simulink model "PMSM_PLL0707"  (R2018b)
settings: Solver=ode45  StartTime=0.0  StopTime=15  FixedStep=Ts  RelTol=1e-4  EnableMultiTasking=on
InitFcn:
  | Ts = 1e-5;
  | Tsample = 1e-3;
  | 
  | Rs = 0.8975;
  | Ld = 1.5e-3;
  | Lq = 1.5e-3;
  | Pn = 3;
  | flux = 0.1764;
  | 
  | Kp_PLL = 1500;
  | Ki_PLL = 1000;
undefined symbols (not defined in the file): DiscIntNeverNeededParam
libraries: powerlib x5, powerlib_extras x2, simulink x1
settings Model: Creator=SUN  LastModifiedBy=liangjin
settings SolverCC: ZeroCrossControl=DisableAll
settings DataIOCC: LimitDataPoints=on  SaveFormat=Array
settings OptimizationCC: ExpressionDepthLimit=2147483647  InitFltsAndDblsToZero=on  LifeSpan=inf
settings DebuggingCC: UnderspecifiedInitializationDetection=Classic  MergeDetectMultiDrivingBlocksExec=none  SolverPrmCheckMsg=warning  FcnCallInpInsideContextMsg=warning  StateNameClashWarn=warning  SFUnexpectedBacktrackingDiag=warning  SFNoUnconditionalDefaultTransitionDiag=warning  SFExecutionAtInitializationDiag=none
settings HardwareCC: ProdBitPerPointer=32  ProdBitPerSizeT=32  ProdBitPerPtrDiffT=32  ProdLargestAtomicFloat=None  ProdIntDivRoundTo=Undefined  ProdEndianess=Unspecified  ProdWordSize=32  ProdHWDeviceType=32-bit Generic
settings ModelReferenceCC: PropagateSignalLabelsOutOfModel=off
settings SFSimCC: SimUseLocalCustomCode=off
settings RTWCC: RTWUseLocalCustomCode=off
settings CodeAppCC: StateflowObjectComments=on
settings GRTTargetCC: TargetLangStandard=C89/C90 (ANSI)  GeneratePreprocessorConditionals=Disable all  CombineOutputUpdateFcns=off  GRTInterface=on
settings ConfigComp: CovMetricSettings=dw  CovHtmlReporting=on  CovSaveCumulativeToWorkspaceVar=on  CovSaveSingleToWorkspaceVar=on  CovExternalEMLEnable=off  CovSFcnEnable=off
settings SimscapeCC: SimscapeNormalizeSystem=off

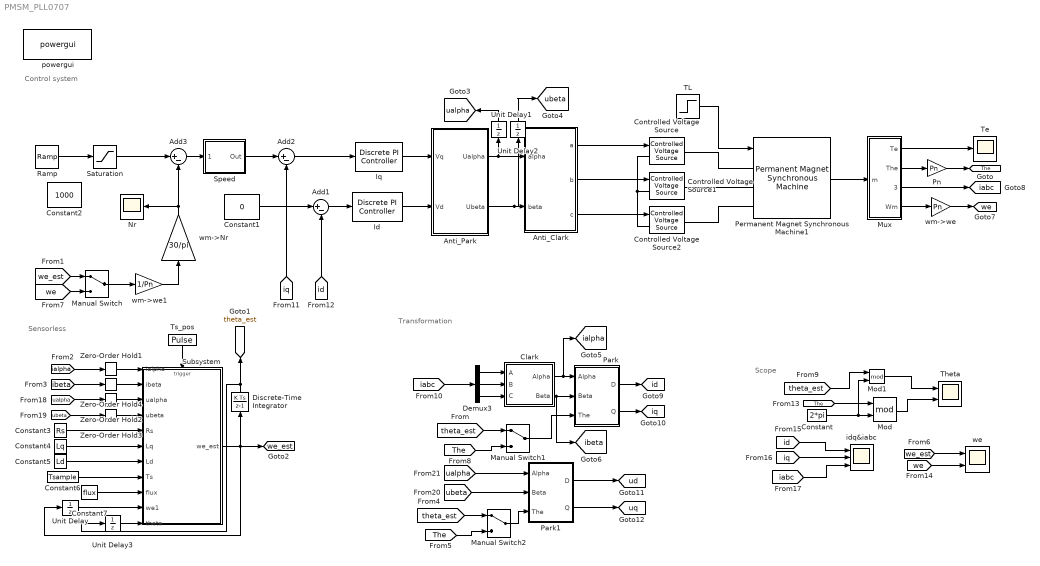
== system PMSM_PLL0707 ==
  note: Scope
  note: Control system
  note: Transformation
  note: Sensorless
  Add1 : Sum  Inputs=|+-
  Add2 : Sum  Inputs=|+-
  Add3 : Sum  Inputs=|+-
  Anti_Clark : Subsystem
  Anti_Park : Subsystem
  Clark : Subsystem
  Constant : Constant  Value=2*pi
  Constant1 : Constant  Value=0
  Constant2 : Constant  Value=1000
  Constant3 : Constant  Value=Rs
  Constant4 : Constant  Value=Lq
  Constant5 : Constant  Value=Ld
  Constant6 : Constant  Value=Tsample
  Constant7 : Constant  Value=flux
  Controlled Voltage Source : powerlib/Electrical Sources/Controlled Voltage Source  Initialize=on  Source_Type=AC  Amplitude=0  Phase=0  Frequency=0  Measurements=None
      settings: SourceProductName=Simscape Electrical
  Controlled Voltage Source1 : powerlib/Electrical Sources/Controlled Voltage Source  Initialize=on  Source_Type=AC  Amplitude=0  Phase=0  Frequency=0  Measurements=None
      settings: SourceProductName=Simscape Electrical
  Controlled Voltage Source2 : powerlib/Electrical Sources/Controlled Voltage Source  Initialize=on  Source_Type=AC  Amplitude=0  Phase=0  Frequency=0  Measurements=None
      settings: SourceProductName=Simscape Electrical
  Demux3 : Demux  Outputs=3
  Discrete-Time Integrator : DiscreteIntegrator  gainval=1  SampleTime=Ts  ICPrevOutput=DiscIntNeverNeededParam  ICPrevScaledInput=DiscIntNeverNeededParam
  Id : powerlib_extras/Discrete  Control Blocks/Discrete PI Controller  Kp=Ld*376  Ki=Rs*376  Par_Limits=[311*0.9*sqrt(1/3) -311*0.9*sqrt(1/3)]  Init=0  Ts=Ts*10
  Iq : powerlib_extras/Discrete  Control Blocks/Discrete PI Controller  Kp=Lq*376  Ki=Rs*376  Par_Limits=[311*0.9*sqrt(1/3) -311*0.9*sqrt(1/3)]  Init=0  Ts=Ts*10
  Manual Switch : ManualSwitch
  Manual Switch1 : ManualSwitch
  Manual Switch2 : ManualSwitch
  Mod : Math  Operator=mod  SaturateOnIntegerOverflow=on
  Mod1 : Math  Operator=mod  SaturateOnIntegerOverflow=on
  Mux : Subsystem
  Nr : Scope
  Park : Subsystem
  Park1 : Subsystem
  Permanent Magnet Synchronous Machine1 : powerlib/Machines/Permanent Magnet Synchronous Machine  NbPhases=3  FluxDistribution=Sinusoidal  RotorType=Salient-pole  MechanicalLoad=Torque Tm  PresetModel=No  ShowDetailedParameters=on  MeasurementBus=off  Resistance=0.8975  Inductance=8.5e-3  dqInductances=[1.5e-3,1.5e-3]  La=0.000835  MachineConstant=Flux linkage established by magnets (V.s)  Flux=0.1764  VoltageCst=95.9863  TorqueCst=0.7938  Flat=120  Mechanical=[0.000311 0.0000001 3]  PolePairs=3  InitialConditions=[0,0, 0,0]  InitialConditions5ph=[0 0 0 0 0 0]  TsPowergui=0  TsBlock=-1  RefAngle=Aligned with phase A axis (original Park)
  Pn : Gain  Gain=Pn
  Ramp : simulink/Sources/Ramp  slope=500  start=0  InitialOutput=0
  Saturation : Saturate  UpperLimit=1000  LowerLimit=-1000
  Speed : Subsystem  AncestorBlock=|  DialogController=POWERSYS.PowerSysDialog  mask(Discrete PI Controller){Kpw=0.01, Kiw=0.01*50, Ba=0, Par_Limits=[80 -80], Init=0, Ts=100*Ts}
      | powerlib_extras/Discrete 
      | Control Blocks/Discrete
      | PI Controller
      mask prompts: Kpw "Proportional gain (Kp):"; Kiw "Integral gain (Ki):"; Ba "feedback gain (Ba)"; Par_Limits "Output limits: [ Upper   Lower ]"; Init "Output initial value:"; Ts "Sample time:"
      mask help: This block implements a discrete PI controller.
      mask init:
      | UpperLimit=Par_Limits(1);
      | LowerLimit=Par_Limits(2);
      | power_initmask();
      mask Help: This block is part of a subset of blocks in the Extras library that does not have documentation associated with it, other than the block mask description.
      mask Display: disp('PI');
  Subsystem : Subsystem
  TL : Step  Time=0  After=0  SampleTime=Ts
  Te : Scope
  Theta : Scope  NumInputPorts=2
  Ts_pos : DiscretePulseGenerator  PulseType=Time based  Period=1e-3  PulseWidth=50
  Unit Delay : UnitDelay  SampleTime=-1
  Unit Delay1 : UnitDelay  SampleTime=10*Ts
  Unit Delay2 : UnitDelay  SampleTime=10*Ts
  Unit Delay3 : UnitDelay  SampleTime=-1
  Zero-Order Hold{1..4} (4 alike) : ZeroOrderHold  SampleTime=10*Ts
  idq&iabc : Scope  NumInputPorts=3
  powergui : powerlib/powergui  SimulationMode=Discrete  SampleTime=Ts  frequency=60  Iterations=50  frequencyindice=0  Pbase=100e6  ErrMax=1e-4  UnitsV=kV  UnitsW=MW  buscounter=0  FunctionMessages=off  echomessages=off  EnableUseOfTLC=off  CurrentSourceSwitches=off  DisableSnubberDevices=off  DisableRonSwitches=off  DisableVfSwitches=off  DisplayEquations=off  SolverType=Tustin/Backward Euler (TBE)  Interpol=off  ExternalGateDelay=off  methode=off  Ts=100  x0status=blocks  SPID=off  SwTol=0  HookPort=off  RestoreLinks=warning  ResistiveCurrentMeasurement=off  Frange=[0:2:500]  Ylog=off  Xlog=on  ShowGrid=off  save=off  variable=ZData  structure=0  ZoomFFT=on  StartTime=0.0  cycles=1  DisplayStyle=1  fundamental=60  FreqAxis=off  MaxFrequency=1000  frequencyindicesteady=1  RmsSteady=1  display=off
  we : Scope  NumInputPorts=2
  wm->Nr : Gain  Gain=30/pi
  wm->we : Gain  Gain=Pn
  wm->we1 : Gain  Gain=1/Pn
  tag scope: The=global, iabc=global, ialpha=global, ibeta=global, id=global, iq=global, theta_est=global, ualpha=global, ubeta=global, ud=global, uq=global, we=global, we_est=global
  wires:
  TL/1 -> Permanent Magnet Synchronous Machine1/1
  Permanent Magnet Synchronous Machine1/1 -> Mux/1(m)
  Add3/1 -> Speed/1(Error)
  Constant1/1 -> Add1/1
  Add1/1 -> Id/1
  wm->Nr/1 -> Add3/2, Nr/1
  Add2/1 -> Iq/1
  Mux/1(Te) -> Te/1
  Mux/2(The) -> Pn/1
  Pn/1 -> [The]
  Mux/4(Wm) -> wm->we/1
  Mux/3(Iabc) -> [iabc]
  Clark/1(Alpha) -> [ialpha], Park/1(Alpha)
  Demux3/1 -> Clark/1(A)
  Demux3/2 -> Clark/2(B)
  Demux3/3 -> Clark/3(C)
  Clark/2(Beta) -> Park/2(Beta), [ibeta]
  Iq/1 -> Anti_Park/1(Vq)
  Id/1 -> Anti_Park/2(Vd)
  Anti_Clark/1(a) -> Controlled Voltage Source/1
  Anti_Clark/2(b) -> Controlled Voltage Source1/1
  Anti_Clark/3(c) -> Controlled Voltage Source2/1
  Speed/1(Out) -> Add2/1
  Constant/1 -> Mod/2, Mod1/2
  Mod/1 -> Theta/2
  wm->we/1 -> [we]
  Ramp/1 -> Saturation/1
  wm->we1/1 -> wm->Nr/1
  Anti_Park/1(Ualpha) -> Unit Delay1/1, Anti_Clark/1(alpha)
  Anti_Park/2(Ubeta) -> Unit Delay2/1, Anti_Clark/2(beta)
  [we_est] -> we/1
  [we_est] -> Manual Switch/1
  [we] -> Manual Switch/2
  [theta_est] -> Manual Switch1/1
  Manual Switch1/1 -> Park/3(The)
  [The] -> Manual Switch1/2
  Saturation/1 -> Add3/1
  [iabc] -> Demux3/1
  Park/1(D) -> [id]
  Park/2(Q) -> [iq]
  [The] -> Mod/1
  [we] -> we/2
  [id] -> idq&iabc/1
  [iq] -> idq&iabc/2
  [iabc] -> idq&iabc/3
  [id] -> Add1/2
  [iq] -> Add2/2
  Manual Switch/1 -> wm->we1/1
  [ualpha] -> Zero-Order Hold2/1
  [ubeta] -> Zero-Order Hold3/1
  [ialpha] -> Zero-Order Hold1/1
  [ibeta] -> Zero-Order Hold4/1
  [The] -> Manual Switch2/2
  Manual Switch2/1 -> Park1/3(The)
  [theta_est] -> Manual Switch2/1
  [ubeta] -> Park1/2(Beta)
  [ualpha] -> Park1/1(Alpha)
  Park1/1(D) -> [ud]
  Park1/2(Q) -> [uq]
  Unit Delay1/1 -> [ualpha]
  Unit Delay2/1 -> [ubeta]
  Discrete-Time Integrator/1 -> [theta_est], Unit Delay3/1
  Subsystem/1(we_est) -> Discrete-Time Integrator/1, [we_est], Unit Delay/1
  Zero-Order Hold1/1 -> Subsystem/1(ialpha)
  Zero-Order Hold4/1 -> Subsystem/2(ibeta)
  Zero-Order Hold2/1 -> Subsystem/3(ualpha)
  Zero-Order Hold3/1 -> Subsystem/4(ubeta)
  Constant3/1 -> Subsystem/5(Rs)
  Constant4/1 -> Subsystem/6(Lq)
  Constant5/1 -> Subsystem/7(Ld)
  Constant6/1 -> Subsystem/8(Ts)
  Constant7/1 -> Subsystem/9(flux)
  Unit Delay/1 -> Subsystem/10(we1)
  Ts_pos/1 -> Subsystem/Trigger
  Unit Delay3/1 -> Subsystem/11(theta)
  [theta_est] -> Mod1/1
  Mod1/1 -> Theta/1
  connections:
  Controlled Voltage Source/LConn1 -- Controlled Voltage Source2/LConn1 -- Controlled Voltage Source1/LConn1
  Controlled Voltage Source/RConn1 -- Permanent Magnet Synchronous Machine1/LConn1
  Controlled Voltage Source1/RConn1 -- Permanent Magnet Synchronous Machine1/LConn2
  Controlled Voltage Source2/RConn1 -- Permanent Magnet Synchronous Machine1/LConn3

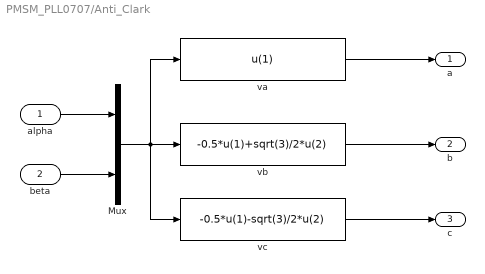
== system PMSM_PLL0707/Anti_Clark ==
  alpha : Inport
  beta : Inport  Port=2
  Mux : Mux  Inputs=2
  va : Fcn  Expr=u(1)
  vb : Fcn  Expr=-0.5*u(1)+sqrt(3)/2*u(2)
  vc : Fcn  Expr=-0.5*u(1)-sqrt(3)/2*u(2)
  a : Outport
  b : Outport  Port=2
  c : Outport  Port=3
  wires:
  va/1 -> a/1
  beta/1 -> Mux/2
  alpha/1 -> Mux/1
  Mux/1 -> vc/1, vb/1, va/1
  vb/1 -> b/1
  vc/1 -> c/1

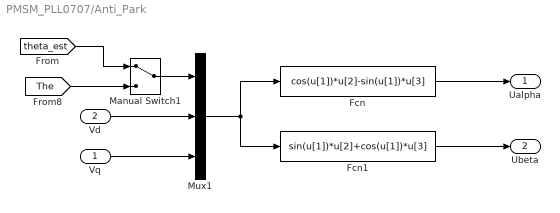
== system PMSM_PLL0707/Anti_Park ==
  Vq : Inport
  Vd : Inport  Port=2
  Fcn : Fcn  Expr=cos(u[1])*u[2]-sin(u[1])*u[3]
  Fcn1 : Fcn  Expr=sin(u[1])*u[2]+cos(u[1])*u[3]
  Manual Switch1 : ManualSwitch
  Mux1 : Mux  Inputs=3
  Ualpha : Outport
  Ubeta : Outport  Port=2
  wires:
  Fcn1/1 -> Ubeta/1
  Fcn/1 -> Ualpha/1
  Mux1/1 -> Fcn/1, Fcn1/1
  Vd/1 -> Mux1/2
  Vq/1 -> Mux1/3
  Manual Switch1/1 -> Mux1/1
  [The] -> Manual Switch1/2
  [theta_est] -> Manual Switch1/1

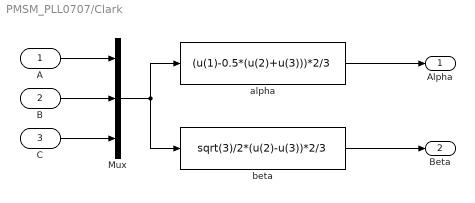
== system PMSM_PLL0707/Clark ==
  A : Inport
  B : Inport  Port=2
  C : Inport  Port=3
  Mux : Mux  Inputs=3
  alpha : Fcn  Expr=(u(1)-0.5*(u(2)+u(3)))*2/3
  beta : Fcn  Expr=sqrt(3)/2*(u(2)-u(3))*2/3
  Alpha : Outport
  Beta : Outport  Port=2
  wires:
  alpha/1 -> Alpha/1
  B/1 -> Mux/2
  C/1 -> Mux/3
  A/1 -> Mux/1
  Mux/1 -> beta/1, alpha/1
  beta/1 -> Beta/1

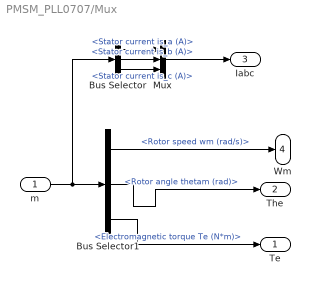
== system PMSM_PLL0707/Mux ==
  m : Inport
  Bus Selector : BusSelector  OutputSignals=Stator current is_a (A),Stator current is_b (A),Stator current is_c (A)
  Bus Selector1 : BusSelector  OutputSignals=Rotor speed wm (rad/s),Rotor angle thetam (rad),Electromagnetic torque Te (N*m)
  Mux : Mux  Inputs=3
  Te : Outport
  The : Outport  Port=2
  Iabc : Outport  Port=3
  Wm : Outport  Port=4
  wires:
  Bus Selector1/1 -> Wm/1  "<Rotor speed wm (rad/s)>"
  Bus Selector1/2 -> The/1  "<Rotor angle thetam (rad)>"
  Bus Selector1/3 -> Te/1  "<Electromagnetic torque Te (N*m)>"
  m/1 -> Bus Selector/1, Bus Selector1/1
  Bus Selector/2 -> Mux/2  "<Stator current is_b (A)>"
  Bus Selector/3 -> Mux/3  "<Stator current is_c (A)>"
  Bus Selector/1 -> Mux/1  "<Stator current is_a (A)>"
  Mux/1 -> Iabc/1

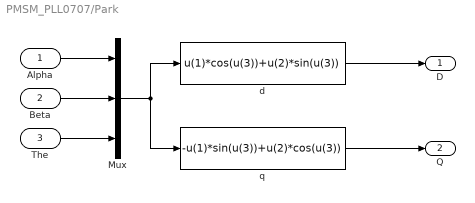
== system PMSM_PLL0707/Park ==
  Alpha : Inport
  Beta : Inport  Port=2
  The : Inport  Port=3
  Mux : Mux  Inputs=3
  d : Fcn  Expr=u(1)*cos(u(3))+u(2)*sin(u(3))
  q : Fcn  Expr=-u(1)*sin(u(3))+u(2)*cos(u(3))
  D : Outport
  Q : Outport  Port=2
  wires:
  d/1 -> D/1
  Beta/1 -> Mux/2
  Alpha/1 -> Mux/1
  Mux/1 -> q/1, d/1
  q/1 -> Q/1
  The/1 -> Mux/3

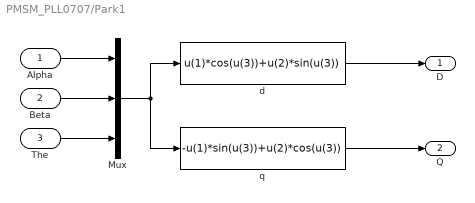
== system PMSM_PLL0707/Park1 ==
  Alpha : Inport
  Beta : Inport  Port=2
  The : Inport  Port=3
  Mux : Mux  Inputs=3
  d : Fcn  Expr=u(1)*cos(u(3))+u(2)*sin(u(3))
  q : Fcn  Expr=-u(1)*sin(u(3))+u(2)*cos(u(3))
  D : Outport
  Q : Outport  Port=2
  wires:
  d/1 -> D/1
  Beta/1 -> Mux/2
  Alpha/1 -> Mux/1
  Mux/1 -> q/1, d/1
  q/1 -> Q/1
  The/1 -> Mux/3

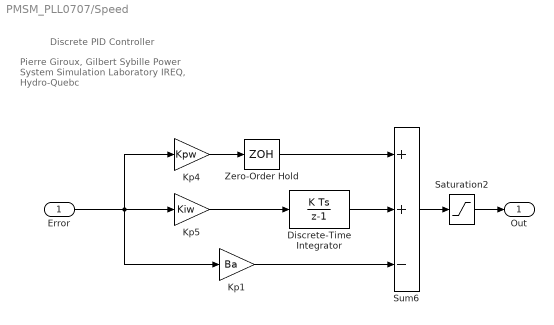
== system PMSM_PLL0707/Speed ==
  note: Discrete PID Controller
  note: Pierre Giroux, Gilbert Sybille
      | Power System Simulation Laboratory
      | IREQ, Hydro-Quebc
  Error : Inport  SampleTime=Ts
  Discrete-Time Integrator : DiscreteIntegrator  InitialCondition=Init  SampleTime=Ts  LimitOutput=on  UpperSaturationLimit=UpperLimit  LowerSaturationLimit=LowerLimit  ICPrevOutput=DiscIntNeverNeededParam  ICPrevScaledInput=DiscIntNeverNeededParam
  Kp1 : Gain  Gain=Ba  SampleTime=Ts  SaturateOnIntegerOverflow=on  OutDataTypeStr=Inherit: Same as input  ParamDataTypeStr=Inherit: Same as input
  Kp4 : Gain  Gain=Kpw  SampleTime=Ts  SaturateOnIntegerOverflow=on  OutDataTypeStr=Inherit: Same as input  ParamDataTypeStr=Inherit: Same as input
  Kp5 : Gain  Gain=Kiw  SampleTime=Ts  SaturateOnIntegerOverflow=on  OutDataTypeStr=Inherit: Same as input  ParamDataTypeStr=Inherit: Same as input
  Saturation2 : Saturate  UpperLimit=UpperLimit  LowerLimit=LowerLimit  SampleTime=Ts
  Sum6 : Sum  Inputs=++-  SampleTime=Ts  SaturateOnIntegerOverflow=on  InputSameDT=on  OutDataTypeStr=Inherit: Same as first input
  Zero-Order Hold : ZeroOrderHold  SampleTime=Ts
  Out : Outport  SampleTime=Ts  InitialOutput=0
  wires:
  Error/1 -> Kp1/1, Kp5/1, Kp4/1
  Zero-Order Hold/1 -> Sum6/1
  Saturation2/1 -> Out/1
  Discrete-Time Integrator/1 -> Sum6/2
  Kp4/1 -> Zero-Order Hold/1
  Kp5/1 -> Discrete-Time Integrator/1
  Sum6/1 -> Saturation2/1
  Kp1/1 -> Sum6/3

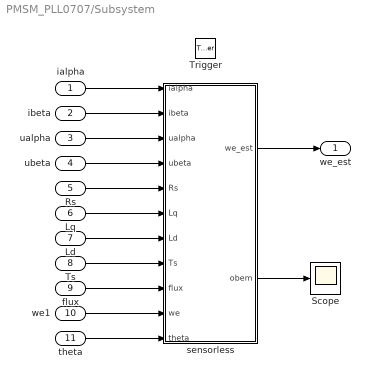
== system PMSM_PLL0707/Subsystem ==
  ialpha : Inport
  ibeta : Inport  Port=2
  ualpha : Inport  Port=3
  ubeta : Inport  Port=4
  Rs : Inport  Port=5
  Lq : Inport  Port=6
  Ld : Inport  Port=7
  Ts : Inport  Port=8
  flux : Inport  Port=9
  we1 : Inport  Port=10
  theta : Inport  Port=11
  Trigger : TriggerPort  VariantControl=Variant  PortDimensions=1
  Scope : Scope
  sensorless : MATLAB Function  TreatAsAtomicUnit=on
  we_est : Outport
  wires:
  ualpha/1 -> sensorless/3(ualpha)
  Ts/1 -> sensorless/8(Ts)
  flux/1 -> sensorless/9(flux)
  ialpha/1 -> sensorless/1(ialpha)
  sensorless/1(we_est) -> we_est/1
  Lq/1 -> sensorless/6(Lq)
  ubeta/1 -> sensorless/4(ubeta)
  ibeta/1 -> sensorless/2(ibeta)
  Rs/1 -> sensorless/5(Rs)
  Ld/1 -> sensorless/7(Ld)
  we1/1 -> sensorless/10(we)
  theta/1 -> sensorless/11(theta)
  sensorless/2(obem) -> Scope/1

== matlab function PMSM_PLL0707/Subsystem/sensorless ==
  data: ialpha input; we_est output; ibeta input; ualpha input; ubeta input; Rs input; Lq input; Ld input; Ts input; flux input; we input; theta input; obem output
function [we_est, obem]  = sensorless(ialpha,ibeta,ualpha,ubeta,Rs,Lq,Ld,Ts,flux,we,theta)

persistent id2 iq2 delta_id delta_iq bemf we1 flag;

if isempty(id2)
    id2=0;iq2=0;delta_id=0;delta_iq=0;bemf=0;we1=0;flag=0;obem=0;
end
ud= cos(theta)*ualpha+sin(theta)*ubeta;
uq=-sin(theta)*ualpha+cos(theta)*ubeta;
id1= cos(theta)*ialpha+sin(theta)*ibeta;
iq1=-sin(theta)*ialpha+cos(theta)*ibeta;

if(bemf < 0)
    flag = 1;
end

we1 = we1+0.715*(we-we1);
temp1 = ud-id2*Rs;
temp1 = temp1+we1*Lq*iq2;
temp1 = temp1*Ts/Ld + id2;
delta_id = delta_id+0.125*((temp1-id1)-delta_id);

temp2 = uq-iq2*Rs;
temp2 = temp2-we1*Ld*id2;
temp2 = temp2-bemf;
temp2 = Ts*iq2/Lq+iq2;
delta_iq = delta_iq+0.5*((temp2-iq1)-delta_iq);

bemf = bemf+delta_iq*Lq/Ts;
if(flag)
    we_est = (bemf+delta_id*Ld/Ts)/flux;
else
    we_est = (bemf-delta_id*Ld/Ts)/flux;
end
obem = bemf;
id2 = id1;
iq2 = iq1;
